simulink model "chap2_11sim"  (Simulink 6.3)
settings: Solver=ode45  StartTime=0.0  StopTime=5  RelTol=1e-3
values from neighbouring files (symbols this model uses):
  kd = 10    [chap2_12int.m]    (also in chap2_12save.mat = 9.99804334002; chap2_4tuning.m = kp*pi/(4*wm); chap2_5tuning.m = kp*pi/(4*wm); chap2_8ctrl.m = -19)
  ki = 0.10    (= 0.1)    [chap2_12int.m]    (also in chap2_12save.mat = 0.0698139131399; chap2_4tuning.m = kp*wm/pi; chap2_5tuning.m = kp*wm/pi)
  kp = 1    [chap2_12int.m]    (also in chap2_12save.mat = 1.01140093599; chap2_4tuning.m = 0.6*km; chap2_5tuning.m = 0.6*km; chap2_8ctrl.m = 9)
libraries: simulink_extras x1
settings Model: LastModifiedBy=Administrator  ExtModeTrigMode=oneshot  ExtModeArmWhenConnect=off  StrictBusMsg=None
settings DataIOCC: LimitDataPoints=off  SignalLoggingName=sigsOut
settings OptimizationCC: BooleanDataType=off
settings DebuggingCC: SolverPrmCheckMsg=none
settings HardwareCC: TargetUnknown=on

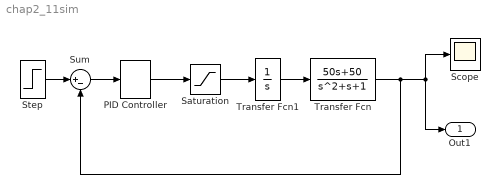
== system chap2_11sim ==
  PID Controller : simulink_extras/Additional Linear/PID Controller  P=kp  I=ki  D=kd
  Saturation : Saturate  UpperLimit=5  LowerLimit=-5
  Scope : Scope
      settings: MaxDataPoints=500000
  Step : Step  Time=0  SampleTime=0
  Sum : Sum  Inputs=|+-  SaturateOnIntegerOverflow=on  InputSameDT=on
  Transfer Fcn : TransferFcn  Numerator=[50 50]  Denominator=[1 1 1]
  Transfer Fcn1 : TransferFcn  Denominator=[1 0]
  Out1 : Outport
  wires:
  Sum/1 -> PID Controller/1
  Step/1 -> Sum/1
  Transfer Fcn/1 -> Sum/2, Scope/1, Out1/1
  PID Controller/1 -> Saturation/1
  Transfer Fcn1/1 -> Transfer Fcn/1
  Saturation/1 -> Transfer Fcn1/1
